simulink model "IntelligentBinPickingGemini"  (R2026a)
settings: Solver=FixedStepAuto  StopTime=200  FixedStep=0.05/5
PreLoadFcn:
  | robotSimParams;
model workspace (MAT data in the model file):
  SL_ROS_VariableLengthArrays_MaxSizes.CommonInfo.ArrayTruncateAction = 'EmitWarning'
  SL_ROS_VariableLengthArrays_MaxSizes.MsgTypeMap = containers.Map
  SL_ROS_VariableLengthArrays_MaxSizes.MsgTypeMap.serialization.keys = {'sensor_msgs/Image', 'sensor_msgs/PointCloud2'}
  SL_ROS_VariableLengthArrays_MaxSizes.MsgTypeMap.serialization.values{1}(1).PropertyName = 'Data'
  SL_ROS_VariableLengthArrays_MaxSizes.MsgTypeMap.serialization.values{1}(1).DataType = 'uint8'
  SL_ROS_VariableLengthArrays_MaxSizes.MsgTypeMap.serialization.values{1}(1).MaxLength = 921600
  SL_ROS_VariableLengthArrays_MaxSizes.MsgTypeMap.serialization.values{1}(2).PropertyName = 'Encoding'
  SL_ROS_VariableLengthArrays_MaxSizes.MsgTypeMap.serialization.values{1}(2).DataType = 'uint8'
  SL_ROS_VariableLengthArrays_MaxSizes.MsgTypeMap.serialization.values{1}(2).MaxLength = 128
  SL_ROS_VariableLengthArrays_MaxSizes.MsgTypeMap.serialization.values{2}(1).PropertyName = 'Data'
  SL_ROS_VariableLengthArrays_MaxSizes.MsgTypeMap.serialization.values{2}(1).DataType = 'uint8'
  SL_ROS_VariableLengthArrays_MaxSizes.MsgTypeMap.serialization.values{2}(1).MaxLength = 9830400
  SL_ROS_VariableLengthArrays_MaxSizes.MsgTypeMap.serialization.values{2}(2).PropertyName = 'Fields'
  SL_ROS_VariableLengthArrays_MaxSizes.MsgTypeMap.serialization.values{2}(2).DataType = 'sensor_msgs/PointField'
  SL_ROS_VariableLengthArrays_MaxSizes.MsgTypeMap.serialization.values{2}(2).MaxLength = 16
  SL_ROS_VariableLengthArrays_MaxSizes.MsgTypeMap.serialization.uniformity = 0
  SL_ROS_VariableLengthArrays_MaxSizes.MsgTypeMap.serialization.keyType = 'char'
  SL_ROS_VariableLengthArrays_MaxSizes.MsgTypeMap.serialization.valueType = 'any'
values from neighbouring files (symbols this model uses):
  MaxDetections = maxObjectDetection    [robotSimParams.m]
  targetEnv = TargetEnvs.Sim3d    [robotSimParams.m]
undefined symbols (not defined in the file or in its folder): binCenterPosition, GeminiERPlan, GeminiERVerify, isSingleDetection, maxVisionObjects, motionPlannerCmdInitValue, posTargetError, robotCommandInitValue
libraries: GeminiRobotics x2
settings Model: Creator=The MathWorks, Inc.  LastModifiedBy=smaddina
settings DebuggingCC: SubsystemReferenceDiagnosticForUnitTest=warning

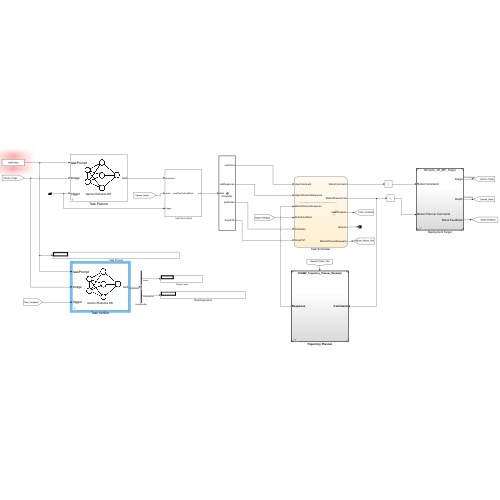
[thumbnail: Simulink's stored preview of the top-level diagram]
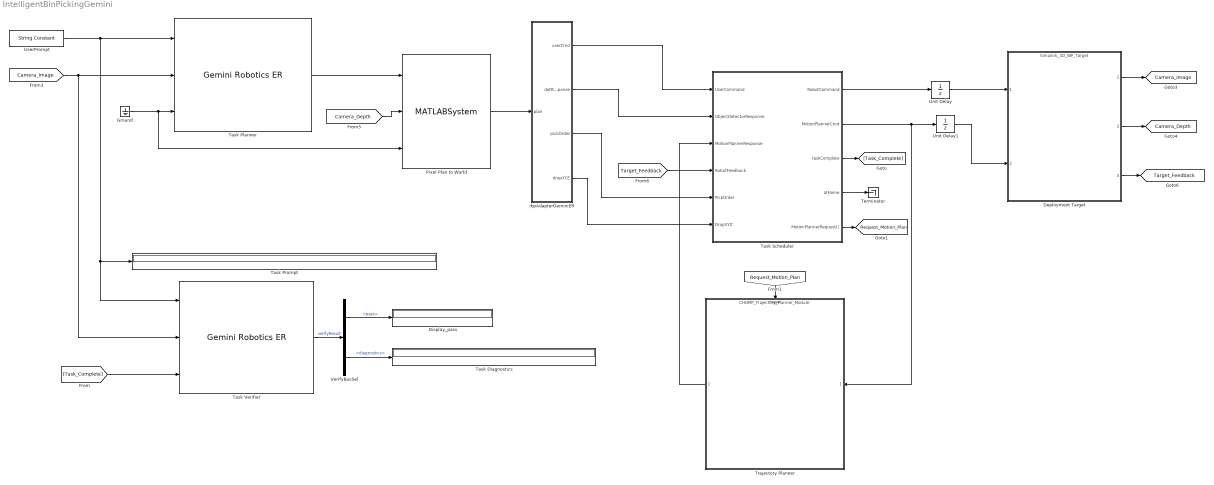
== system IntelligentBinPickingGemini ==
  Deployment Target : ModelReference  ModelNameDialog=Simulink_3D_IBP_Target  SimulationMode=Normal  ModelReferenceVersion=7.8
  Display_pass : Display
  Ground : Ground
  Pixel Plan to World : MATLABSystem  System=pixelPlanToWorldBlock  FocalLength=750  PrincipalPoint=[640 360]  CameraLoc=[0.5 0 1.5]  CameraRot=pi/2*ones([1 3])  MaxBinDistance=0.95  DropHeightOffset=0.1  RobotOffsetZ=0.625001  MaxDetections=8
      mask Type: pixelPlanToWorldBlock
  Task Diagnostics : Display
  Task Planner : GeminiRobotics/Gemini Robotics ER  UseEnvApiKey=on  ApiKey=[]  Mode=GeminiERPlan('MaxDetections', MaxDetections)  ScenarioPrompt=|  ThinkingBudget=0  SampleTime=inf
      | You are guiding a robot arm that performs intelligent bin picking.
      | 
      | Scene layout (overhead camera looking straight down):
      | - A rectangular bin in the centre of the image holds unsorted white plastic pipe fittings.
      | - A flat work table to the LEFT of the bin is a placement target.
      | - A flat work table to the RIGHT of the bin is a placement target.
      | - A robot arm (may appear at the image edges) performs the pick-and-place.
      | 
      | The objects in the bin are white plastic pipe fittings of four types:
      | - Cross fitting  (X-shape): four-way connector, four symmetric arms in a plus pattern.
      | - Tee fitting    (T-shape): three-way connector, one straight channel with one perpendicular branch.
      | - Elbow fitting  (L-shape): two-way connector bent 90 degrees.
      | - Straight fitting (I-shape): cylindrical straight-through connector, no bends.
      link override Sys: Task=PlanTask()
  Task Prompt : Display
  Task Scheduler : Stateflow chart  TreatAsAtomicUnit=on
  Task Verifier : GeminiRobotics/Gemini Robotics ER  UseEnvApiKey=on  ApiKey=[]  Mode=GeminiERVerify()  ScenarioPrompt=|  ThinkingBudget=0  SampleTime=inf
      | You are guiding a robot arm that performs intelligent bin picking.
      | 
      | Scene layout (overhead camera looking straight down):
      | - A rectangular bin in the centre of the image holds unsorted white plastic pipe fittings.
      | - A flat work table to the LEFT of the bin is a placement target.
      | - A flat work table to the RIGHT of the bin is a placement target.
      | - A robot arm (may appear at the image edges) performs the pick-and-place.
      | 
      | The objects in the bin are white plastic pipe fittings of four types:
      | - Cross fitting  (X-shape): four-way connector, four symmetric arms in a plus pattern.
      | - Tee fitting    (T-shape): three-way connector, one straight channel with one perpendicular branch.
      | - Elbow fitting  (L-shape): two-way connector bent 90 degrees.
      | - Straight fitting (I-shape): cylindrical straight-through connector, no bends.
      link override Sys: Task=VerifyTask()
  Terminator : Terminator
  Trajectory Planner : ModelReference  ModelNameDialog=CHOMP_Trajectory_Planner_Module.slx  SimulationMode=Normal  ModelReferenceVersion=7.6  TriggerPortName=function  TriggerPortTriggerType=function-call  TriggerPortStatesWhenEnabling=held
  Unit Delay : UnitDelay  SampleTime=-1
  Unit Delay1 : UnitDelay  SampleTime=-1
  UserPrompt : StringConstant  String=taskPrompt
  VerifyBusSel : BusSelector  OutputSignals=pass,diagnostics
  ibpAdapterGeminiER : MATLAB Function  TreatAsAtomicUnit=on
  tag scope: Camera_Depth=global, Camera_Image=global, Request_Motion_Plan=global, Target_Feedback=global
  wires:
  Task Scheduler/5(MotionPlannerRequest()) -> [Request_Motion_Plan]
  [Request_Motion_Plan] -> Trajectory Planner/Trigger
  Task Scheduler/2(MotionPlannerCmd) -> Unit Delay1/1, Trajectory Planner/1
  Task Scheduler/1(RobotCommand) -> Unit Delay/1
  Unit Delay/1 -> Deployment Target/1
  Unit Delay1/1 -> Deployment Target/2
  Deployment Target/1 -> [Camera_Image]
  Deployment Target/2 -> [Camera_Depth]
  Deployment Target/3 -> [Target_Feedback]
  [Target_Feedback] -> Task Scheduler/4(RobotFeedback)
  Trajectory Planner/1 -> Task Scheduler/3(MotionPlannerResponse)
  ibpAdapterGeminiER/2(detResponse) -> Task Scheduler/2(ObjectDetectorResponse)
  ibpAdapterGeminiER/3(pickOrder) -> Task Scheduler/5(PickOrder)
  ibpAdapterGeminiER/4(dropXYZ) -> Task Scheduler/6(DropXYZ)
  ibpAdapterGeminiER/1(userCmd) -> Task Scheduler/1(UserCommand)
  UserPrompt/1 -> Task Verifier/1, Task Prompt/1, Task Planner/1
  Ground/1 -> Pixel Plan to World/3, Task Planner/3
  Task Planner/1 -> Pixel Plan to World/1
  [Camera_Depth] -> Pixel Plan to World/2
  Pixel Plan to World/1 -> ibpAdapterGeminiER/1(plan)
  [Camera_Image] -> Task Verifier/2, Task Planner/2
  VerifyBusSel/1 -> Display_pass/1  "<pass>"
  VerifyBusSel/2 -> Task Diagnostics/1  "<diagnostics>"
  [Task_Complete] -> Task Verifier/3
  Task Verifier/1 -> VerifyBusSel/1  "verifyResult"
  Task Scheduler/3(taskComplete) -> [Task_Complete]
  Task Scheduler/4(atHome) -> Terminator/1

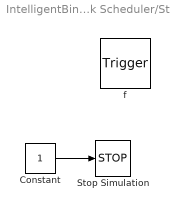
== system IntelligentBinPickingGemini/Task Scheduler/Stop ==
  f : TriggerPort  TriggerType=function-call  VariantControl=(inherit)
      settings: CopyFcn=Stateflow.SLINSF.SimulinkMan.removeBlockPreDeleteFcn  PreDeleteFcn=Stateflow.SLINSF.SimulinkMan.unsafePredeleteFcn
  Constant : Constant
  Stop Simulation : Stop
  wires:
  Constant/1 -> Stop Simulation/1

== matlab function IntelligentBinPickingGemini/ibpAdapterGeminiER ==
  data: userCmd output Bus: BUS_user_command size=1; plan input Bus: geminiTaskPlannerBus; detResponse output Bus: BUS_object_detector_response size=1; pickOrder output int32 size=[1, MaxDetections]; dropXYZ output double size=[MaxDetections, 3]; MaxDetections parameter
function [userCmd, detResponse, pickOrder, dropXYZ] = PlanAdapter(plan, MaxDetections)
%#codegen
% Convert geminiTaskPlannerBus to IBP Task Scheduler inputs.
N_LIT = 8;  % fixed literal for struct allocation — must match MaxDetections
N     = int32(MaxDetections);
cnt   = min(N, int32(plan.count));

emptyObj = struct('Name',         zeros(1,256,'uint8'), ...
                  'Type',         zeros(1,256,'uint8'), ...
                  'AttachBody',   zeros(1,256,'uint8'), ...
                  'Radius',       0.0, ...
                  'Length',       0.0, ...
                  'Color',        zeros(1,3), ...
                  'Opacity',      0.0, ...
                  'Displacement', zeros(3,1), ...
                  'EulAnglesZYX', zeros(3,1), ...
                  'ObjectPos',    zeros(3,1), ...
                  'ObjectEulZYX', zeros(3,1), ...
                  'PickPos',      zeros(3,1), ...
                  'PickEulZYX',   zeros(3,1), ...
                  'ID',           ObjectTypesID.Unknown);

detResponse = struct('Status', int32(-1), 'NumObjects', uint32(0), 'MaxNumObjects', uint32(N_LIT), 'Objects', repmat(emptyObj, N_LIT, 1));
if cnt > int32(0)
    detResponse.Status     = int32(1);
    detResponse.NumObjects = uint32(cnt);
    for i = 1:cnt
        detResponse.Objects(i).PickPos    = plan.world_xyz(i,:)';
        detResponse.Objects(i).PickEulZYX = [0; pi; 0];
        detResponse.Objects(i).ID         = ObjectTypesID.Unknown;
        detResponse.Objects(i).ObjectPos  = plan.world_xyz(i,:)';
    end
end

userCmd = struct('Mode', PickAndPlaceModes.PickAll, 'PickSelectedObjectID', ObjectTypesID.Unknown, 'PickAllOrder', ObjectTypesID.Unknown, 'Enable', true, 'Reset', false);
userCmd.Enable       = true;
userCmd.Mode         = PickAndPlaceModes.PickAll;
userCmd.PickAllOrder = ObjectTypesID.Unknown;

pickOrder = int32(plan.pick_order(1:N_LIT))';
dropXYZ   = plan.drop_xyz(1:N_LIT, :);

== stateflow chart IntelligentBinPickingGemini/Task Scheduler ==
  state Stop [function]
  state Setup
    entry:
    ii = 1;
    obsObjectCounter = 1;
    MotionPlannerCmd = motionPlannerCmdInitValue;
    RobotCommand = robotCommandInitValue;
    pickAllObjectIndex = uint32(1);
    objectToPickIndex  = uint32(0);
    objectPickedIndices = zeros(1,maxVisionObjects);
    isVacuumOn = false;
    SimFailed = false;
    atHome = false;
  state DeactivateVacuum
    entry:
    disp('Sending Deactivate Vacuum Command');
    RobotCommand.CommandToProcess = int32(enumCmd.deactivate_vacuum);
    RobotCommand.ProcessCommand = true;
    exit:
    RobotCommand.ProcessCommand = false;
    isVacuumOn = false;
  state SendToHome
    entry:
    disp('Sending robot to home position');
    success = false;
    atHome = true;
    RobotCommand.CommandToProcess = int32(enumCmd.send_to_home);
    RobotCommand.ProcessCommand = true;
    if targetEnv == TargetEnvs.Sim3d
    success = true;
    end
    during:
    if ~success
    % To make the robot motion non-blocking and vizualize in Sim3d
    [posErr, orErr] = calcTaskSE3MaxError(homePoseCartesian, RobotFeedback.TooltipTransform);
    if posErr < posTargetError
    success = true;
    end
    end
    exit:
    RobotCommand.ProcessCommand = false;
    atHome = false;
  state DetectObjects
    state ExtractObjectToPickSingleDetection
      en:
      motionCmdWithCollisionObjects = addCollisionObjectsInfo(ObjectDetectorResponse);
      generateDroppingPoses(ObjectDetectorResponse);
      [isObjectInScene, objectToPickPos, objectToPickEul, objectToPickIndex, pickAllObjectIndex] = getObjectToPick(UserCommand, ObjectDetectorResponse, pickAllObjectIndex);
    (junction 417) -> ExtractObjectToPickSingleDetection [order 1] : [ObjectDetectorResponse.NumObjects >= 1]
    ExtractObjectToPickSingleDetection -> (junction 438) [order 2] : [isObjectInScene == true]
  state StopSimulation
    entry:
    objectPickedIndices = zeros(1, maxVisionObjects);
    Stop();
    taskComplete = true;
  state GoToPickingPose
    state GetPickingTrajectoryFromMotionPlanner
      entry:
      % Here based on object Pos and Eul get picking pose
      pickPos = objectToPickPos + [0.0; 0.0; 0.01];  % Bring the arm to 1cm above the pick position
      pickEul = objectToPickEul;
      %Create a motion planner task bus
      MotionPlannerCmd = createMotionTask(int32(objectToPickIndex), 'Pick', uint32(300), 0.2, RobotFeedback.JointPos, pickPos, objectToPickEul);
      % Add obstacle objects
      MotionPlannerCmd.NumObstacleObjects = ObjectDetectorResponse.NumObjects - 1;
      ii= 1;
      obsObjectCounter = 1;
      for ii = 1:(ObjectDetectorResponse.NumObjects)
      if objectToPickIndex ~= ii
      MotionPlannerCmd.ObstacleObjects(obsObjectCounter) = ObjectDetectorResponse.Objects(ii);
      obsObjectCounter = obsObjectCounter + 1;
      end
      end
      % Send request to motion planner
      MotionPlannerRequest;
    state SendPickingTrajectoryToRobot
      entry:
      % Send trajectory to driver
      disp("Send traj to robot");
      RobotCommand.JointTrajectory = MotionPlannerResponse.JointTrajectory;
      RobotCommand.CommandToProcess = int32(enumCmd.precomputed_joint_trj);
      RobotCommand.ProcessCommand = true;
      posErr = Inf;
      orErr = Inf;
      success = false;
      during:
      RobotCommand.ProcessCommand = false;
      %  Check error and exit when tooltip reaches desired pose.
      T_task = eul2tform(pickEul');
      T_task(1:3,4) = pickPos;
      [posErr, orErr] = calcTaskSE3MaxError(T_task, RobotFeedback.TooltipTransform);
      if posErr < posTargetError
      success = true;
      end
      exit:
    GetPickingTrajectoryFromMotionPlanner -> (junction 14) : [MotionPlannerResponse.RequestID == MotionPlannerCmd.RequestID]
    (junction 14) -> SendPickingTrajectoryToRobot [order 1] : [MotionPlannerResponse.Status == 1 && ...
        | MotionPlannerResponse.IsPosValid == 1 && ...
        | MotionPlannerResponse.IsVelValid == 1 &&...
        |  MotionPlannerResponse.IsAccValid == 1]
  state ActivateVacuum
    entry:
    disp('Sending Activate Vacuum Command');
    RobotCommand.CommandToProcess = int32(enumCmd.activate_vacuum);
    RobotCommand.ProcessCommand = true;
    exit:
    RobotCommand.ProcessCommand = false;
    isVacuumOn = true;
  state GoToDroppingPose
    state RequestDroppingTrajectoryFromMotionPlanner
      entry:
      droppingPose = getDroppingPose(ObjectDetectorResponse,objectToPickIndex,droppingPoses, RobotFeedback.TooltipTransform);
      % Create motion planner task bus
      MotionPlannerCmd = createMotionTask(int32(objectToPickIndex), 'Place', uint32(300), 0.2, RobotFeedback.JointPos, droppingPose(1:3), droppingPose(4:6));
      % Add obstacle objects
      MotionPlannerCmd.NumObstacleObjects = ObjectDetectorResponse.NumObjects - 1;
      ii= 1;
      obsObjectCounter = 1;
      for ii = 1:(ObjectDetectorResponse.NumObjects)
      if objectToPickIndex ~= ii
      MotionPlannerCmd.ObstacleObjects(obsObjectCounter) = ObjectDetectorResponse.Objects(ii);
      obsObjectCounter = obsObjectCounter + 1;
      end
      end
      % Send request to motion planner
      MotionPlannerRequest;
    state SendDroppingTrajectoryToRobot
      entry:
      % Send trajectory to driver
      RobotCommand.JointTrajectory = MotionPlannerResponse.JointTrajectory;
      RobotCommand.CommandToProcess = int32(enumCmd.precomputed_joint_trj);
      RobotCommand.ProcessCommand = true;
      posErr = Inf;
      orErr = Inf;
      success = false;
      during:
      RobotCommand.ProcessCommand = false;
      %  Check error and exit when tooltip reaches desired pose.
      T_task = eul2tform(droppingPose(4:6)');
      T_task(1:3,4) = droppingPose(1:3);
      [posErr, orErr] = calcTaskSE3MaxError(T_task, RobotFeedback.TooltipTransform);
      if posErr < posTargetError
      success = true;
      end
      exit:
    RequestDroppingTrajectoryFromMotionPlanner -> (junction 128) : [MotionPlannerResponse.RequestID == MotionPlannerCmd.RequestID]
    (junction 128) -> SendDroppingTrajectoryToRobot [order 1] : [MotionPlannerResponse.Status == 1 && ...
        | MotionPlannerResponse.IsPosValid == 1 && ...
        | MotionPlannerResponse.IsVelValid == 1 && ...
        | MotionPlannerResponse.IsAccValid == 1]
  state MotionPlannerFailed
    en:
    disp('Motion Planner failed');
    SimFailed = true;
  SendPickingTrajectoryToRobot -> ActivateVacuum : [success == true]
  SendToHome -> (junction 417) [order 2] : [success == true]
  (junction 417) -> StopSimulation [order 2] : [ObjectDetectorResponse.NumObjects == 0]{disp('No objects detected. Stopping simulation')}
  ActivateVacuum -> RequestDroppingTrajectoryFromMotionPlanner : {pause(0.5)}
  ExtractObjectToPickSingleDetection -> StopSimulation [order 1] : [objectToPickIndex == uint32(-1)]
      | {disp('No more objects to pick. Stopping simulation')}
  (junction 438) -> GetPickingTrajectoryFromMotionPlanner : {pause(1)}
  (default) -> Setup
  Setup -> (junction 498) : [UserCommand.Enable == true && RobotFeedback.IsValid]
  (junction 498) -> (junction 500) [order 2] : [nnz(objectPickedIndices) == 0]
  (junction 498) -> DeactivateVacuum [order 1] : [nnz(objectPickedIndices) > 0]
  (junction 500) -> SendToHome
  (junction 519) -> DeactivateVacuum [order 1] : [isVacuumOn == true]
  DeactivateVacuum -> SendToHome : {pause(1)}
  SendDroppingTrajectoryToRobot -> (junction 256) : [success == true]
  (junction 519) -> SendToHome [order 2]
  SendToHome -> (junction 532) [order 1] : [SimFailed == true]
  (junction 532) -> StopSimulation : {disp('Stopping simulation')}
  (junction 128) -> MotionPlannerFailed [order 2]
  (junction 256) -> (junction 485)
  (junction 14) -> MotionPlannerFailed [order 2]
  MotionPlannerFailed -> (junction 527)
  (junction 485) -> (junction 527)
  (junction 527) -> (junction 535)
  (junction 535) -> (junction 253)
  (junction 253) -> (junction 519)
  data: userCommandIn function_input Bus: BUS_user_command size=1; objectDetectorResponseIn function_input Bus: BUS_object_detector_response size=1; isObjectInSceneOut function_output; objectToPickPosOut function_output double size=[3 1]; objectToPickEulOut function_output double size=[3 1]; objectToPickIndexOut function_output uint32 size=1; pickAllObjectIndexOut function_output uint32 size=1; pickAllObjectIndexIn function_input uint32 size=1; detectorResponse function_input; motionCmd function_output; objectDetectorResponse function_input; droppingPoseOut function_output double size=[6 1]; ObjectDetectorResponseIn function_input Bus: BUS_object_detector_response size=1; objectToPickIdx function_input; droppingPosesIn function_input size=[6, maxVisionObjects]; unused function_input; requestIDIn function_input; typeIn function_input; maxIterationsIn function_input; sampleTimeIn function_input; q0In function_input; targetPosIn function_input; targetEulIn function_input; motionPlannerCmdOut function_output; T_aIn function_input double size=[4 4]; T_bIn function_input double size=[4 4]; posErrOut function_output double size=1; orErrOut function_output double size=1; RobotCommand output Bus: BUS_robot_command size=1; UserCommand input Bus: BUS_user_command size=1; ObjectDetectorResponse input Bus: BUS_object_detector_response size=1; MotionPlannerResponse input Bus: BUS_motion_planner_response size=1; MotionPlannerCmd output Bus: BUS_motion_planner_cmd size=1; isObjectInScene local boolean size=1 =false; objectToPickEul local; objectToPickPos local; ii local uint32 size=1; obsObjectCounter local uint32 size=1; RobotFeedback input Bus: BUS_robot_feedback size=1; T_task local double size=[4, 4]; orErr local double size=1; posErr local double size=1; posTargetError parameter double size=1; droppingPoses local double size=[6, maxVisionObjects] =zeros(6, maxVisionObjects); pickEul local double size=[3 1]; pickPos local double size=[3 1]; pickAllObjectIndex local uint32 size=1; objectToPickIndex local uint32 size=1; droppingPose local double size=[6 1]; robotCommandInitValue parameter size=1; isSingleDetection parameter; binCenterPosition parameter; objectPickedIndices local double size=[1 maxVisionObjects] =zeros(1, maxVisionObjects); targetEnv parameter; motionCmdWithCollisionObjects local Bus: BUS_motion_planner_cmd size=1; success local; maxVisionObjects parameter double size=1; isVacuumOn local boolean size=1 =false; SimFailed local boolean size=1 =false; motionPlannerCmdInitValue parameter size=1; homePoseCartesian local =homePoseCartesian; PickOrder input int32 size=[1, maxVisionObjects]; DropXYZ input double size=[maxVisionObjects, 3]; taskComplete output boolean; atHome output boolean
  events: MotionPlannerRequest output FUNCTION_CALL_EVENT
  function [isObjectInSceneOut, objectToPickPosOut, objectToPickEulOut, objectToPickIndexOut, pickAllObjectIndexOut] = getObjectToPick(userCommandIn, objectDetectorResponseIn, pickAllObjectIndexIn):
    | function [isObjectInSceneOut, objectToPickPosOut, objectToPickEulOut, objectToPickIndexOut, pickAllObjectIndexOut] = getObjectToPick(userCommandIn, objectDetectorResponseIn, pickAllObjectIndexIn)
    | 
    | isObjectInSceneOut = false;
    | objectToPickPosOut = zeros(3,1);
    | objectToPickEulOut = zeros(3,1);
    | objectToPickIndexOut = uint32(0);
    | pickAllObjectIndexOut = pickAllObjectIndexIn;
    | 
    | if isSingleDetection
    |     partsToPickGT = zeros(objectDetectorResponseIn.NumObjects - nnz(objectPickedIndices), 6);
    |     if ~isempty(partsToPickGT)
    |         partsToPickGTIdx = int32(1);
    |         partsToPickDetectedIdx = zeros(1,10);
    |         for ii = 1:objectDetectorResponseIn.NumObjects
    |             if ~any(objectPickedIndices == ii)
    |                 partsToPickGT(partsToPickGTIdx, 1:3) = objectDetectorResponseIn.Objects(ii).PickPos;
    |                 partsToPickGT(partsToPickGTIdx, 4) = objectDetectorResponseIn.Objects(ii).PickEulZYX(1);
    |                 partsToPickDetectedIdx(partsToPickGTIdx) = double(ii);
    |                 partsToPickGTIdx = partsToPickGTIdx + int32(1);
    |             end
    |         end
    | 
    |         bestPriority = int32(2147483647);
    |         partIDToPick = int32(0);
    |         for jj = 1:size(partsToPickGT, 1)
    |             detIdx = int32(partsToPickDetectedIdx(jj));
    |             if detIdx > int32(0) && PickOrder(detIdx) < bestPriority
    |                 bestPriority = PickOrder(detIdx);
    |                 partIDToPick = int32(jj);
    |             end
    |         end
    | 
    |         if partIDToPick > int32(0)
    |             isObjectInSceneOut = true;
    |             objectToPickPosOut = partsToPickGT(partIDToPick, 1:3)';
    |             objectToPickIndexOut = uint32(partsToPickDetectedIdx(partIDToPick));
    |             objectToPickEulOut = [0; pi; 0];
    |             if pickAllObjectIndexIn < length(userCommandIn.PickAllOrder)
    |                 pickAllObjectIndexOut = pickAllObjectIndexIn + uint32(1);
    |             else
    |                 pickAllObjectIndexOut = uint32(1);
    |             end
    |             if size(partsToPickGT, 1) == objectDetectorResponseIn.NumObjects
    |                 objectPickedIndices(1) = double(objectToPickIndexOut);
    |             else
    |                 objectPickedIndices(nnz(objectPickedIndices) + 1) = double(objectToPickIndexOut);
    |             end
    |         end
    |     else
    |         objectToPickIndexOut = uint32(0);
    |     end
    | 
    | else
    |     partsToPickGT = zeros(objectDetectorResponseIn.NumObjects, 6);
    |     if ~isempty(partsToPickGT)
    |         for ii = 1:objectDetectorResponseIn.NumObjects
    |             partsToPickGT(ii, 1:3) = objectDetectorResponseIn.Objects(ii).PickPos;
    |             partsToPickGT(ii, 4) = objectDetectorResponseIn.Objects(ii).PickEulZYX(1);
    |         end
    | 
    |         bestPriority = int32(2147483647);
    |         partIDToPick = int32(0);
    |         for jj = 1:objectDetectorResponseIn.NumObjects
    |             if PickOrder(jj) < bestPriority
    |                 bestPriority = PickOrder(jj);
    |                 partIDToPick = int32(jj);
    |             end
    |         end
    | 
    |         if partIDToPick > int32(0)
    |             isObjectInSceneOut = true;
    |             objectToPickPosOut = partsToPickGT(partIDToPick, 1:3)';
    |             objectToPickEulOut = [0; pi; 0];
    |             objectToPickIndexOut = uint32(partIDToPick);
    |             if pickAllObjectIndexIn < length(userCommandIn.PickAllOrder)
    |                 pickAllObjectIndexOut = pickAllObjectIndexIn + uint32(1);
    |             else
    |                 pickAllObjectIndexOut = uint32(1);
    |             end
    |             if isempty(find(objectPickedIndices,1))
    |                 objectPickedIndices(1) = double(partIDToPick);
    |             else
    |                 objectPickedIndices(nnz(objectPickedIndices) + 1) = double(partIDToPick);
    |             end
    |         end
    |     else
    |         objectToPickIndexOut = uint32(0);
    |     end
    | end
  function motionCmd = addCollisionObjectsInfo(detectorResponse):
    | function motionCmd = addCollisionObjectsInfo(detectorResponse)
    | 
    | motionCmd = motionPlannerCmdInitValue;
    | 
    | numObjectsToPick = detectorResponse.NumObjects;
    | motionCmd.NumObstacleObjects = numObjectsToPick;
    | 
    | for ii = 1:numObjectsToPick
    |    motionCmd.ObstacleObjects(ii) = detectorResponse.Objects(ii);
    | end
    | 
    | 
    | end
  function generateDroppingPoses(objectDetectorResponse):
    | function generateDroppingPoses(objectDetectorResponse)
    |  
    | %% Define dropping poses
    | 
    | 
    | %For single detection workflow, the dropping poses will get defined once
    | %and then used in the getDroppingPoses method.
    | 
    | %For multiple detections, ensure that the dropping poses get generated only
    | %once. Check the presence of non-zero value in objectPickedIndices to
    | %detect subsequent detections.
    | 
    | %In this implementation, the user defined drop POSITION doesn't change based
    | %on the pose of the object before picking. However, the orientation of the object
    | %may change during the course of picking other objects and that is taken
    | %into account in the getDroppingPose method.
    | 
    | %Generate dropping pose only once
    | if isempty(find(objectPickedIndices,1))
    |     numOfParts = objectDetectorResponse.NumObjects;
    |     droppingPoses = zeros(6, maxVisionObjects);
    |     for i=1:numOfParts
    |         if i>numOfParts-1
    |             droppingPoses(:, i) = [0.01 0.59 -0.018 0 pi 0]';
    |         else
    |             droppingPoses(:, i) = [0.01+(double(i)-1)*0.07 0.75 -0.018 0 pi 0]';
    |         end
    |     end
    | end
  function droppingPoseOut = getDroppingPose(ObjectDetectorResponseIn,objectToPickIdx,droppingPosesIn,~):
    | function droppingPoseOut = getDroppingPose(ObjectDetectorResponseIn,objectToPickIdx,droppingPosesIn,~)
    | % Use Gemini drop_xyz when available; fall back to generateDroppingPoses for detection-only prompts.
    | droppingPoseOut = droppingPosesIn(:,objectToPickIdx);
    | if any(DropXYZ(objectToPickIdx, :))
    |     droppingPoseOut(1:3) = DropXYZ(objectToPickIdx, :)';
    |     droppingPoseOut(4) = 0;
    | end
  function motionPlannerCmdOut = createMotionTask(requestIDIn, typeIn, maxIterationsIn, sampleTimeIn, q0In, targetPosIn, targetEulIn):
    | function motionPlannerCmdOut = createMotionTask(requestIDIn, typeIn, maxIterationsIn, sampleTimeIn, q0In, targetPosIn, targetEulIn)
    | 
    | % In this one I didn't expose the max velocity because the planner doesn't
    | % consider the acceleration limits directly. We use a conservative Lin and
    | % Ang limits to control acceleration.
    | 
    | % q0In = [q0In; 0; 0; 0; 0; 0; 0;];
    | 
    | % Initialize bus
    | motionPlannerCmdOut = motionCmdWithCollisionObjects;
    | 
    | % Configure motion planner tasks
    | motionPlannerCmdOut.RequestID = requestIDIn;
    | motionPlannerCmdOut.NumTasks = uint32(4);
    | motionPlannerCmdOut.MaxIterations = maxIterationsIn;
    | motionPlannerCmdOut.SampleTime = sampleTimeIn;
    | motionPlannerCmdOut.InitialPositions = q0In;
    | % Task 1: End effector pose
    | motionPlannerCmdOut.Tasks(1).Name(1:length(uint8('TooltipTaskSE3'))) = uint8('TooltipTaskSE3');
    | motionPlannerCmdOut.Tasks(1).Type(1:length(typeIn))  = uint8(typeIn);
    | motionPlannerCmdOut.Tasks(1).FrameName(1:length(uint8('Bellow')))  = uint8('Bellow');
    | motionPlannerCmdOut.Tasks(1).p = targetPosIn;
    | motionPlannerCmdOut.Tasks(1).eulZYX = targetEulIn;
    | motionPlannerCmdOut.Tasks(1).MaxLinVel = 0.10;  % 0.072 0.1 0.15
    | motionPlannerCmdOut.Tasks(1).MaxAngVel = 0.4;    % 0.4
    | motionPlannerCmdOut.Tasks(1).Weight = 1.0;
    | motionPlannerCmdOut.Tasks(1).MaxLinError = 0.01;        % 0.01
    | motionPlannerCmdOut.Tasks(1).MaxAngError = deg2rad(2);  % 2
  function [posErrOut,orErrOut] = calcTaskSE3MaxError(T_aIn, T_bIn):
    | function [posErrOut,orErrOut] = calcTaskSE3MaxError(T_aIn, T_bIn)
    |  
    | % Position error is max of coordinate
    | posErrOut = max(abs(T_aIn(1:3,4) - T_bIn(1:3,4)));
    | 
    | % Orientation error with quaternions. Also using max for error
    | q_a = tform2quat(T_aIn);
    | q_b = tform2quat(T_bIn);
    | 
    | % skew
    | S_a = [      0, -q_a(4),  q_a(3); 
    |         q_a(4),       0, -q_a(2); 
    |        -q_a(3),  q_a(2),       0];
    |     
    | or_error = q_b(1)*q_a(2:4)'-q_a(1)*q_b(2:4)'- S_a*q_b(2:4)';    % q = [w x y z]
    | 
    | orErrOut = max(abs(or_error));
